simulink model "archivoAuxiliarPractica4_0"  (R2021b)
settings: Solver=ode45  StartTime=0.0  StopTime=60  RelTol=1e-3
undefined symbols (not defined in the file): a1, a2, a3, a4, a5, a6, b0, b1, b2, b3, b4, b5, K, Radio, Rf, ro
libraries: simulink x5
settings Model: Creator=jualc  LastModifiedBy=jualc
settings SolverCC: MaxConsecutiveMinStep=1000

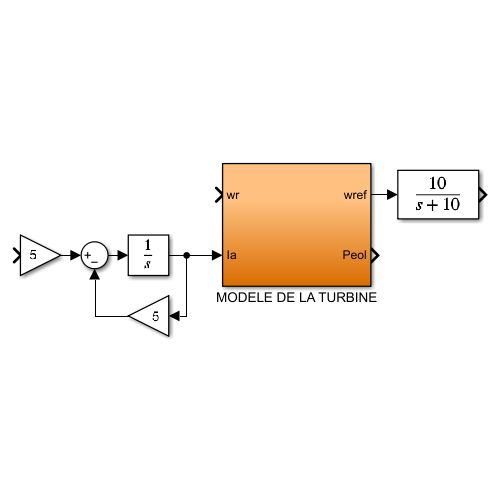
[thumbnail: Simulink's stored preview of the top-level diagram]
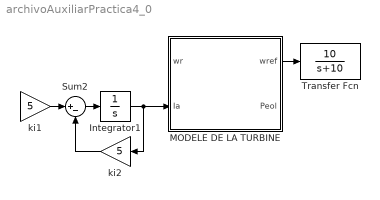
== system archivoAuxiliarPractica4_0 ==
  Integrator1 : Integrator  InitialCondition=30
  MODELE DE LA TURBINE : Subsystem
  Sum2 : Sum  Inputs=|+-
  Transfer Fcn : TransferFcn  Numerator=[10]  Denominator=[1 10]
  ki1 : Gain  Gain=5
  ki2 : Gain  Gain=5
  wires:
  MODELE DE LA TURBINE/1(wref) -> Transfer Fcn/1
  Integrator1/1 -> ki2/1, MODELE DE LA TURBINE/2(Ia)
  Sum2/1 -> Integrator1/1
  ki1/1 -> Sum2/1
  ki2/1 -> Sum2/2

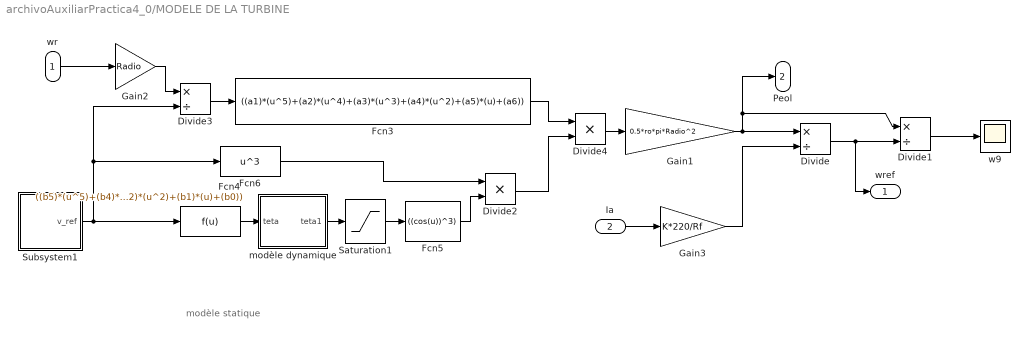
== system archivoAuxiliarPractica4_0/MODELE DE LA TURBINE ==
  note: modèle statique
  wr : Inport
  Ia : Inport  Port=2
  Divide : Product  Inputs=*/
  Divide1 : Product  Inputs=*/
  Divide2 : Product  Inputs=**
  Divide3 : Product  Inputs=*/
  Divide4 : Product  Inputs=**
  Fcn3 : Fcn  Expr=((a1)*(u^5)+(a2)*(u^4)+(a3)*(u^3)+(a4)*(u^2)+(a5)*(u)+(a6))
  Fcn4 : Fcn  Expr=((b5)*(u^5)+(b4)*(u^4)+(b3)*(u^3)+(b2)*(u^2)+(b1)*(u)+(b0))
  Fcn5 : Fcn  Expr=((cos(u))^3)
  Fcn6 : Fcn  Expr=u^3
  Gain1 : Gain  Gain=0.5*ro*pi*Radio^2
  Gain2 : Gain  Gain=Radio
  Gain3 : Gain  Gain=K*220/Rf
  Saturation1 : Saturate  UpperLimit=0.095  LowerLimit=0
  Subsystem1 : Subsystem
  modèle dynamique : Subsystem
  w9 : Scope
  wref : Outport  VectorParamsAs1DForOutWhenUnconnected=off
  Peol : Outport  Port=2  VectorParamsAs1DForOutWhenUnconnected=off
  wires:
  Gain1/1 -> Peol/1, Divide1/1, Divide/1
  Fcn3/1 -> Divide4/1
  Divide/1 -> wref/1, Divide1/2
  Gain3/1 -> Divide/2
  Gain2/1 -> Divide3/1
  Divide3/1 -> Fcn3/1
  Subsystem1/1(v_ref) -> Fcn4/1, Fcn6/1, Divide3/2
  wr/1 -> Gain2/1
  Divide4/1 -> Gain1/1
  Fcn4/1 -> modèle dynamique/1(teta)
  modèle dynamique/1(teta1) -> Saturation1/1
  Fcn5/1 -> Divide2/2
  Fcn6/1 -> Divide2/1
  Divide2/1 -> Divide4/2
  Ia/1 -> Gain3/1
  Saturation1/1 -> Fcn5/1
  Divide1/1 -> w9/1

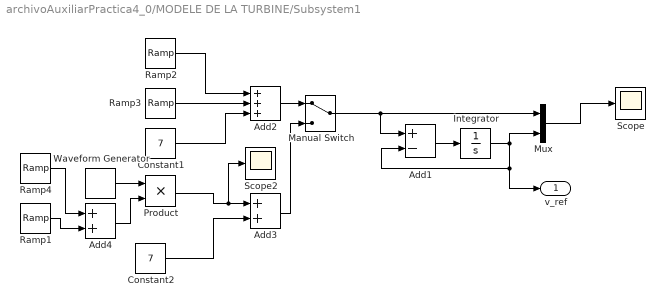
== system archivoAuxiliarPractica4_0/MODELE DE LA TURBINE/Subsystem1 ==
  Add1 : Sum  Inputs=+-
  Add2 : Sum  Inputs=+++
  Add3 : Sum
  Add4 : Sum
  Constant1 : Constant  Value=7
  Constant2 : Constant  Value=7
  Integrator : Integrator  InitialCondition=7  LimitOutput=on  UpperSaturationLimit=10000  LowerSaturationLimit=0
  Manual Switch : ManualSwitch
  Mux : Mux  Inputs=2
  Product : Product
  Ramp1 : simulink/Sources/Ramp  slope=-0.5  start=12  InitialOutput=0
  Ramp2 : simulink/Sources/Ramp  slope=0.5  start=10  InitialOutput=0
  Ramp3 : simulink/Sources/Ramp  slope=-0.5  start=12  InitialOutput=0
  Ramp4 : simulink/Sources/Ramp  slope=0.5  start=10  InitialOutput=0
  Scope : Scope
  Scope2 : Scope
  Waveform Generator : simulink/Sources/Waveform Generator  OutMin=[]  OutMax=[]  OutDataTypeStr=double  SelectedSignal=1  Signals=sin(2,0.3,0)+sin(1.5,0.15,0.1)#  BlockNames=MultiportSwitch_54ba8690b966479#MultiportSwitch_db4e6e1e4f36485  SampleTime=0.1
  v_ref : Outport  VectorParamsAs1DForOutWhenUnconnected=off
  wires:
  Mux/1 -> Scope/1
  Integrator/1 -> v_ref/1, Add1/2, Mux/2
  Add1/1 -> Integrator/1
  Ramp2/1 -> Add2/1
  Ramp3/1 -> Add2/2
  Constant1/1 -> Add2/3
  Manual Switch/1 -> Add1/1, Mux/1
  Add2/1 -> Manual Switch/1
  Constant2/1 -> Add3/2
  Waveform Generator/1 -> Product/1
  Ramp4/1 -> Add4/1
  Ramp1/1 -> Add4/2
  Add4/1 -> Product/2
  Product/1 -> Scope2/1, Add3/1
  Add3/1 -> Manual Switch/2

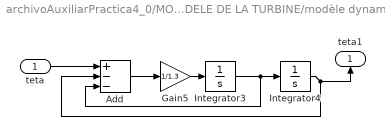
== system archivoAuxiliarPractica4_0/MODELE DE LA TURBINE/modèle dynamique ==
  teta : Inport
  Add : Sum  Inputs=+--
  Gain5 : Gain  Gain=1/1.3
  Integrator3 : Integrator
  Integrator4 : Integrator  InitialCondition=0.0955
  teta1 : Outport  VectorParamsAs1DForOutWhenUnconnected=off
  wires:
  Gain5/1 -> Integrator3/1
  Integrator3/1 -> Add/3, Integrator4/1
  Add/1 -> Gain5/1
  Integrator4/1 -> Add/2, teta1/1
  teta/1 -> Add/1
